simulink model "third_approach_plus_compensation"  (R2020b)
settings: Solver=VariableStepAuto  StartTime=0.0  StopTime=10.0  RelTol=1e-3
libraries: roblocks x4
settings Model: Creator=yrza  LastModifiedBy=User

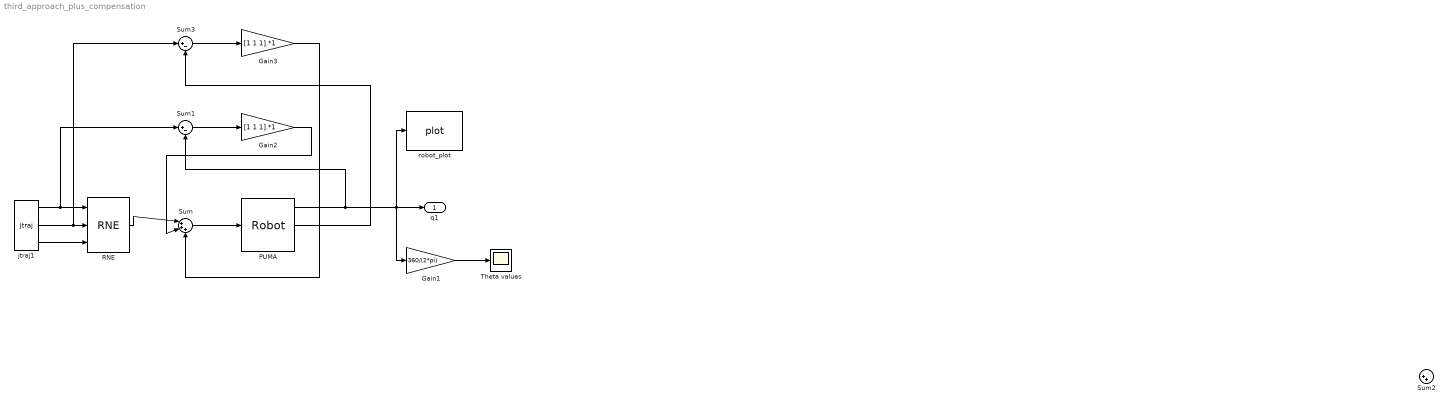
== system third_approach_plus_compensation ==
  Gain1 : Gain  Gain=360/(2*pi)
  Gain2 : Gain  Gain=[1 1 1].*1
  Gain3 : Gain  Gain=[1 1 1].*1
  PUMA : roblocks/Arm/Robot  robot=p560  q0=[0 0 0]
  RNE : roblocks/Arm/RNE  robot=p560  grav=[0 0 9.81]
  Sum : Sum  Inputs=|+++
  Sum1 : Sum  Inputs=|+-
  Sum2 : Sum  Inputs=|++
  Sum3 : Sum  Inputs=|+-
  Theta values : Scope
  jtraj1 : roblocks/Toolbox/jtraj  q0=[0 0 0]  qf=[pi/2 -pi/4 -pi/4]  tmax=2  ts=0.02
  robot_plot : roblocks/Arm/plot  robot=p560  fps=5  holdplot=on
  q1 : Outport
  wires:
  Gain1/1 -> Theta values/1
  jtraj1/1 -> Sum1/1, RNE/1
  RNE/1 -> Sum/1
  Sum/1 -> PUMA/1
  Sum1/1 -> Gain2/1
  Gain2/1 -> Sum/2
  jtraj1/2 -> Sum3/1, RNE/2
  jtraj1/3 -> RNE/3
  PUMA/1 -> Gain1/1, robot_plot/1, q1/1, Sum1/2
  Sum3/1 -> Gain3/1
  Gain3/1 -> Sum/3
  PUMA/2 -> Sum3/2
